simulink model "model_podstawowy_2019b"  (R2020a)
settings: Solver=VariableStepAuto  StartTime=0.0  StopTime=10.0  RelTol=1e-3
undefined symbols (not defined in the file): g, J, L, m, M, Q2
settings Model: Creator=maelstro  LastModifiedBy=maelstro

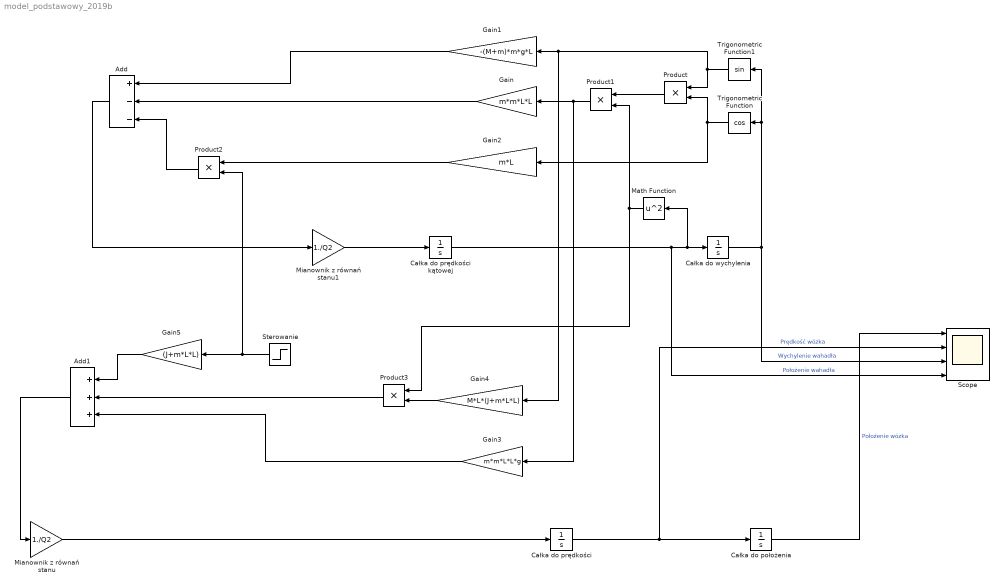
== system model_podstawowy_2019b ==
  Add : Sum  Inputs=+--
  Add1 : Sum  Inputs=+++
  Całka do położenia : Integrator
  Całka do prędkości : Integrator
  Całka do prędkości kątowej : Integrator
  Całka do wychylenia : Integrator
  Gain : Gain  Gain=m*m*L*L
  Gain1 : Gain  Gain=-(M+m)*m*g*L
  Gain2 : Gain  Gain=m*L
  Gain3 : Gain  Gain=m*m*L*L*g
  Gain4 : Gain  Gain=M*L*(J+m*L*L)
  Gain5 : Gain  Gain=(J+m*L*L)
  Math Function : Math  Operator=square  SaturateOnIntegerOverflow=on
  Mianownik z równań stanu : Gain  Gain=1./Q2
  Mianownik z równań stanu1 : Gain  Gain=1./Q2
  Product{,1..3} (4 alike) : Product
  Scope : Scope  NumInputPorts=4
  Sterowanie : Step  SampleTime=0
  Trigonometric Function : Trigonometry  Operator=cos
  Trigonometric Function1 : Trigonometry
  wires:
  Mianownik z równań stanu/1 -> Całka do prędkości/1
  Całka do prędkości/1 -> Scope/2, Całka do położenia/1  "Prędkość wózka"
  Mianownik z równań stanu1/1 -> Całka do prędkości kątowej/1
  Całka do prędkości kątowej/1 -> Scope/4, Math Function/1, Całka do wychylenia/1  "Położenie wahadła"
  Product/1 -> Product1/1
  Math Function/1 -> Product1/2, Product3/1
  Product1/1 -> Gain/1, Gain3/1
  Trigonometric Function1/1 -> Product/1, Gain4/1, Gain1/1
  Trigonometric Function/1 -> Gain2/1, Product/2
  Całka do wychylenia/1 -> Trigonometric Function1/1, Trigonometric Function/1, Scope/3  "Wychylenie wahadła"
  Gain2/1 -> Product2/1
  Sterowanie/1 -> Gain5/1, Product2/2
  Gain1/1 -> Add/1
  Gain/1 -> Add/2
  Product2/1 -> Add/3
  Add/1 -> Mianownik z równań stanu1/1
  Gain4/1 -> Product3/2
  Gain5/1 -> Add1/1
  Product3/1 -> Add1/2
  Gain3/1 -> Add1/3
  Add1/1 -> Mianownik z równań stanu/1
  Całka do położenia/1 -> Scope/1  "Położenie wózka"
